simulink library "utility_lib"  (Simulink 6.3)
undefined symbols (not defined in the file): constants, MACH, quat_IC, subsref
libraries: utility_lib x28, simulink x27
settings Model: LastModifiedBy=E700252  ExtModeAutoUpdateStatusClock=off  StrictBusMsg=None

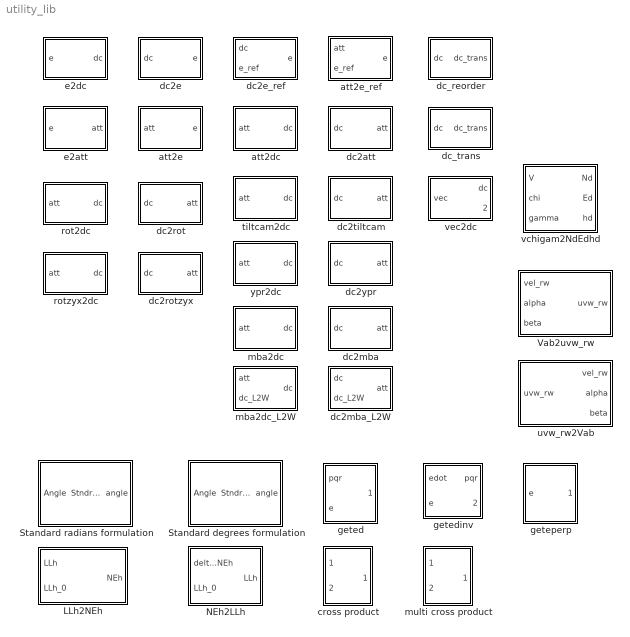
== system utility_lib ==
  LLh2NEh : Subsystem
  NEh2LLh : Subsystem
  Standard degrees formulation : Subsystem
  Standard radians formulation : Subsystem
  Vab2uvw_rw : Subsystem
  att2dc : Subsystem
  att2e : Subsystem  mask{quat_IC=quat_IC}
      mask prompts: quat_IC "quat IC"
  att2e_ref : Subsystem
  cross product : Subsystem
      mask Type: Cross Product
      mask Description: Calculates the cross product of two 3x1 vectors.
      mask Help:
      | <p>This block calculates the cross product of two 3x1 vectors, ie.</p>
      | 
      | <ul>C(1) = A(2)*B(3) - A(3)*B(2)</ul>
      | <ul>C(2) = A(3)*B(1) - A(1)*B(3)</ul>
      | <ul>C(3) = A(1)*B(2) - A(2)*B(1)</ul>
      | 
      | <p>The block inputs and output contain more than one signal as described below.</p>
      | 
      | <p><H4>Block Vector Input 1 - A</H4>
      | <ul>
      | <li>A(1)</li>
      | <li>A(2)</li>
      | <li>A(3)</li>
      | </ul>
      | </p>
      | 
      | <p><H4>Block Vector Input 2 - B</H4>
      | <ul>
      | <li>B(1)</li>
      | <li>B(2)</li>
      | <li>B(3)</li>
      | </ul>
      | </p>
      | 
      | <p><H4>Block Vector Output - Cross Product (AxB)</H4>
      | <ul>
      | <li>C(1)</li>
      | <li>C(2)</li>
      | <li>C(3)</li>
      | </ul>
      | </p>
      mask Display: disp('Cross\nProduct')
  dc2att : Subsystem
  dc2e : Subsystem  mask{quat_IC=quat_IC}
      mask prompts: quat_IC "quat IC"
  dc2e_ref : Subsystem
  dc2mba : Subsystem
  dc2mba_L2W : Subsystem
  dc2rot : Subsystem  mask{rot_order=zyx}
      mask prompts: rot_order "rot order"
      mask init:
      | try
      |     rot_def = {
      |         'zyx',[1 2 3],[1 2 3],1
      |         'yxz',[3 1 2],[2 3 1],1
      |         'xzy',[2 3 1],[3 1 2],1
      |         'xyz',[3 2 1],[3 2 1],-1
      |         'yzx',[1 3 2],[1 3 2],-1
      |         'zxy',[2 1 3],[2 1 3],-1
      |     };
      |     [tf,rot_idx] = ismember(rot_order,rot_def(:,1));
      |     rot_in_order = rot_def{rot_idx,2};
      |     rot_out_order = rot_def{rot_idx,3};
      |     rot_sign = rot_def{rot_idx,4};
      | 
      |     % set_param(gcb,'Tag',rot_order);
      | catch
      |     rethrow(lasterror)
      | end
      mask StyleString: popup(zyx|yxz|xzy|xyz|yzx|zxy)
  dc2rotzyx : Subsystem
  dc2tiltcam : Subsystem
  dc2ypr : Subsystem
  dc_reorder : Subsystem  mask{elements=[1 2 3]}
  dc_trans : Subsystem
  e2att : Subsystem
  e2dc : Subsystem
  geted : Subsystem
  getedinv : Subsystem
  geteperp : Subsystem
  mba2dc : Subsystem
  mba2dc_L2W : Subsystem
  multi cross product : Subsystem
      mask Type: Cross Product
      mask Description: Calculates the pairwise cross product of the columns of two 3xN matrices.
      mask Help:
      | <p>This block calculates the pairwise cross product of the columns of two 3xN matrices., ie.</p>
      | 
      | <ul>C(1,n) = A(2,n)*B(3,n) - A(3,n)*B(2,n)</ul>
      | <ul>C(2,n) = A(3,n)*B(1,n) - A(1,n)*B(3,n)</ul>
      | <ul>C(3,n) = A(1,n)*B(2,n) - A(2,n)*B(1,n)</ul>
      | 
      | <p>The block inputs and output contain more than one signal as described below.</p>
      | 
      | <p><H4>Block Matrix Input 1 - A(3,N)</H4></p>
      | 
      | <p><H4>Block Matrix Input 2 - B(3,N)</H4></p>
      | 
      | <p><H4>Block Matrix Output - C(3,N)</H4> </p>
      mask Display: disp('Multi\nCross\nProduct')
  rot2dc : Subsystem  mask{rot_order=zyx}
      mask prompts: rot_order "rot order"
      mask init: same as utility_lib/dc2rot
      mask StyleString: popup(zyx|yxz|xzy|xyz|yzx|zxy)
  rotzyx2dc : Subsystem
  tiltcam2dc : Subsystem
  uvw_rw2Vab : Subsystem
  vchigam2NdEdhd : Subsystem
  vec2dc : Subsystem
  ypr2dc : Subsystem

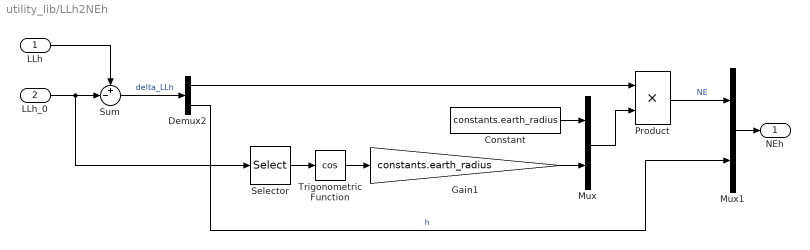
== system utility_lib/LLh2NEh ==
  LLh : Inport
  LLh_0 : Inport  Port=2
  Constant : Constant  Value=constants.earth_radius
  Demux2 : Demux  Outputs=[2 1]
  Gain1 : Gain  Gain=constants.earth_radius  SaturateOnIntegerOverflow=on
  Mux : Mux  Inputs=2
  Mux1 : Mux  Inputs=2
  Product : Product  Inputs=**  SaturateOnIntegerOverflow=on  InputSameDT=on
  Selector : Selector  InputPortWidth=3
  Sum : Sum  Inputs=+-|  SaturateOnIntegerOverflow=on  InputSameDT=on
  Trigonometric Function : Trigonometry  Operator=cos
  NEh : Outport
  wires:
  Trigonometric Function/1 -> Gain1/1
  Mux/1 -> Product/2
  LLh_0/1 -> Selector/1, Sum/2
  Demux2/2 -> Mux1/2  "h"
  Gain1/1 -> Mux/2
  Product/1 -> Mux1/1  "NE"
  Mux1/1 -> NEh/1
  Constant/1 -> Mux/1
  Selector/1 -> Trigonometric Function/1
  Sum/1 -> Demux2/1  "delta_LLh"
  Demux2/1 -> Product/1
  LLh/1 -> Sum/1

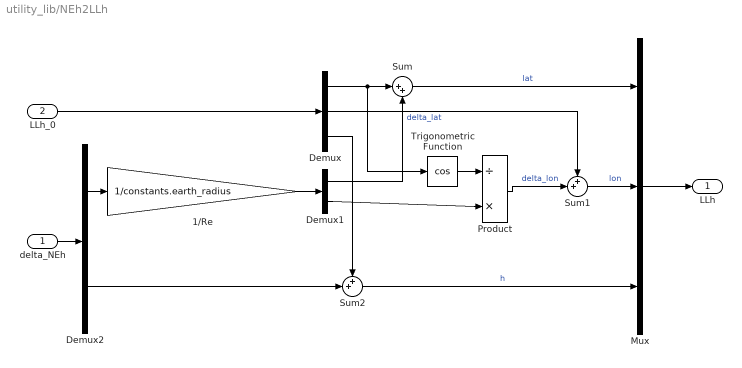
== system utility_lib/NEh2LLh ==
  delta_NEh : Inport
  LLh_0 : Inport  Port=2
  1/Re : Gain  Gain=1/constants.earth_radius  SaturateOnIntegerOverflow=on
  Demux : Demux  Outputs=3
  Demux1 : Demux  Outputs=2
  Demux2 : Demux  Outputs=[2 1]
  Mux : Mux  Inputs=3
  Product : Product  Inputs=/*  SaturateOnIntegerOverflow=on  InputSameDT=on
  Sum : Sum  Inputs=|++  SaturateOnIntegerOverflow=on  InputSameDT=on
  Sum1 : Sum  Inputs=++|  SaturateOnIntegerOverflow=on  InputSameDT=on
  Sum2 : Sum  Inputs=++|  SaturateOnIntegerOverflow=on  InputSameDT=on
  Trigonometric Function : Trigonometry  Operator=cos
  LLh : Outport
  wires:
  Mux/1 -> LLh/1
  Demux2/1 -> 1/Re/1
  Demux1/1 -> Sum/2  "delta_lat"
  Demux/1 -> Sum/1, Trigonometric Function/1
  Demux1/2 -> Product/2
  LLh_0/1 -> Demux/1
  1/Re/1 -> Demux1/1
  Sum/1 -> Mux/1  "lat"
  Trigonometric Function/1 -> Product/1
  Demux/2 -> Sum1/1
  Product/1 -> Sum1/2  "delta_lon"
  Sum1/1 -> Mux/2  "lon"
  delta_NEh/1 -> Demux2/1
  Demux2/2 -> Sum2/2
  Demux/3 -> Sum2/1
  Sum2/1 -> Mux/3  "h"

== system utility_lib/Standard degrees formulation ==
  Angle : Inport
  Constant : Constant  Value=180
  Constant1 : Constant  Value=360
  Constant2 : Constant  Value=180
  Math Function : Math  Operator=mod  SaturateOnIntegerOverflow=on
  Sum : Sum
  Sum1 : Sum  Inputs=+-
  Stndrd  angle : Outport
  wires:
  Constant2/1 -> Sum1/2
  Sum1/1 -> Stndrd  angle/1
  Math Function/1 -> Sum1/1
  Constant1/1 -> Math Function/2
  Constant/1 -> Sum/2
  Angle/1 -> Sum/1
  Sum/1 -> Math Function/1

== system utility_lib/Standard radians formulation ==
  Angle : Inport
  Constant : Constant  Value=pi
  Constant1 : Constant  Value=2*pi
  Constant2 : Constant  Value=pi
  Math Function : Math  Operator=mod  SaturateOnIntegerOverflow=on
  Sum : Sum
  Sum1 : Sum  Inputs=+-
  Stndrd  angle : Outport
  wires:
  Constant2/1 -> Sum1/2
  Sum1/1 -> Stndrd  angle/1
  Math Function/1 -> Sum1/1
  Constant1/1 -> Math Function/2
  Constant/1 -> Sum/2
  Angle/1 -> Sum/1
  Sum/1 -> Math Function/1

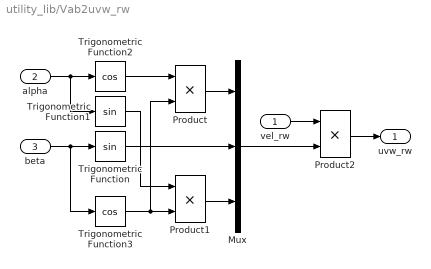
== system utility_lib/Vab2uvw_rw ==
  vel_rw : Inport
  alpha : Inport  Port=2
  beta : Inport  Port=3
  Mux : Mux  Inputs=3
  Product : Product  RndMeth=Zero
  Product1 : Product  RndMeth=Zero
  Product2 : Product  RndMeth=Zero
  Trigonometric Function : Trigonometry
  Trigonometric Function1 : Trigonometry
  Trigonometric Function2 : Trigonometry  Operator=cos
  Trigonometric Function3 : Trigonometry  Operator=cos
  uvw_rw : Outport
  wires:
  alpha/1 -> Trigonometric Function2/1, Trigonometric Function1/1
  beta/1 -> Trigonometric Function3/1, Trigonometric Function/1
  Trigonometric Function2/1 -> Product/1
  Trigonometric Function3/1 -> Product/2, Product1/2
  Trigonometric Function1/1 -> Product1/1
  Trigonometric Function/1 -> Mux/2
  Product1/1 -> Mux/3
  Product/1 -> Mux/1
  Mux/1 -> Product2/2
  vel_rw/1 -> Product2/1
  Product2/1 -> uvw_rw/1

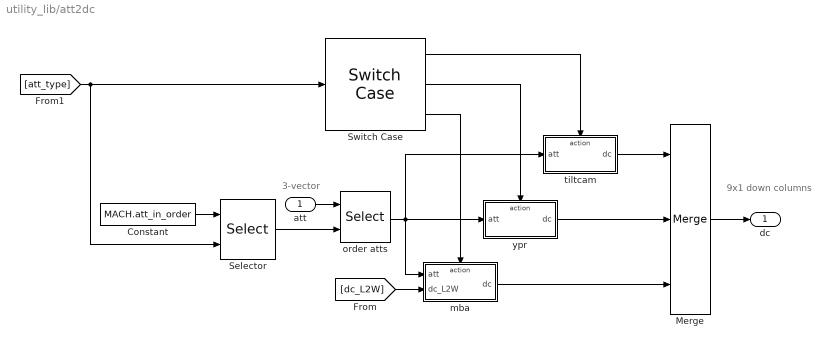
== system utility_lib/att2dc ==
  note: 3-vector
  note: 9x1
      | down columns
  att : Inport
  Constant : Constant  Value=MACH.att_in_order
  Merge : Merge  Inputs=3
  Selector : Selector  InputType=Matrix  Elements=[1 3]  RowSrc=External  Columns=-1  InputPortWidth=3
  Switch Case : SwitchCase  CaseConditions={1, [2 3], [4 5]}  CaseShowDefault=off
  mba : Subsystem  TreatAsAtomicUnit=on
  order atts : Selector  ElementSrc=External  Elements=att_order  InputPortWidth=3
  tiltcam : Subsystem  TreatAsAtomicUnit=on
  ypr : Subsystem  TreatAsAtomicUnit=on
  dc : Outport
  wires:
  order atts/1 -> ypr/1(att), tiltcam/1(att), mba/1(att)
  att/1 -> order atts/1
  Merge/1 -> dc/1
  [att_type] -> Switch Case/1, Selector/2
  tiltcam/1(dc) -> Merge/1
  ypr/1(dc) -> Merge/2
  mba/1(dc) -> Merge/3
  Switch Case/1 -> tiltcam/Action
  Switch Case/2 -> ypr/Action
  Switch Case/3 -> mba/Action
  [dc_L2W] -> mba/2(dc_L2W)
  Selector/1 -> order atts/2
  Constant/1 -> Selector/1

== system utility_lib/att2e ==
  att : Inport  PortDimensions=3
  att2dc : utility_lib/att2dc
  dc2e : utility_lib/dc2e  quat_IC=quat_IC
  e : Outport
  wires:
  att2dc/1 -> dc2e/1
  att/1 -> att2dc/1
  dc2e/1 -> e/1

== system utility_lib/att2e_ref ==
  att : Inport  PortDimensions=3
  e_ref : Inport  Port=2
  att2dc : utility_lib/att2dc
  dc2e_ref : utility_lib/dc2e_ref
  e : Outport
  wires:
  dc2e_ref/1 -> e/1
  att/1 -> att2dc/1
  att2dc/1 -> dc2e_ref/1
  e_ref/1 -> dc2e_ref/2

== system utility_lib/cross product ==
  a(1) a(2) a(3) : Inport
  b(1) b(2) b(3) : Inport  Port=2
  Product : Product  SaturateOnIntegerOverflow=on  RndMeth=Zero  InputSameDT=on
  Product1 : Product  SaturateOnIntegerOverflow=on  RndMeth=Zero  InputSameDT=on
  Selector : Selector  Elements=[2 3 1]  InputPortWidth=3
  Selector1 : Selector  Elements=[3 1 2]  InputPortWidth=3
  Selector2 : Selector  Elements=[2 3 1]  InputPortWidth=3
  Selector3 : Selector  Elements=[3 1 2]  InputPortWidth=3
  Sum : Sum  Inputs=+|-  SaturateOnIntegerOverflow=on  InputSameDT=on
  c(1) c(2) c(3) : Outport  InitialOutput=0
  wires:
  Selector3/1 -> Product1/1
  Selector2/1 -> Product1/2
  Product1/1 -> Sum/2
  Selector1/1 -> Product/2
  Product/1 -> Sum/1
  a(1) a(2) a(3)/1 -> Selector3/1, Selector/1
  Selector/1 -> Product/1
  b(1) b(2) b(3)/1 -> Selector2/1, Selector1/1
  Sum/1 -> c(1) c(2) c(3)/1

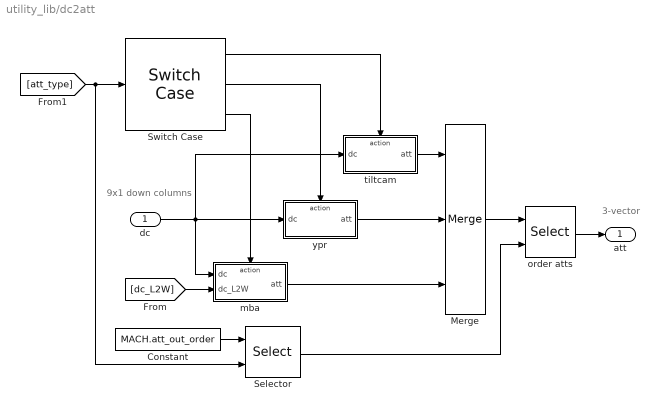
== system utility_lib/dc2att ==
  note: 9x1
      | down columns
  note: 3-vector
  dc : Inport
  Constant : Constant  Value=MACH.att_out_order
  Merge : Merge  Inputs=3
  Selector : Selector  InputType=Matrix  Elements=[1 3]  RowSrc=External  Columns=-1  InputPortWidth=3
  Switch Case : SwitchCase  CaseConditions={1, [2 3], [4 5]}  CaseShowDefault=off
  mba : Subsystem  TreatAsAtomicUnit=on
  order atts : Selector  ElementSrc=External  Elements=att_order  InputPortWidth=3
  tiltcam : Subsystem  TreatAsAtomicUnit=on
  ypr : Subsystem  TreatAsAtomicUnit=on
  att : Outport
  wires:
  [dc_L2W] -> mba/2(dc_L2W)
  Switch Case/2 -> ypr/Action
  Switch Case/1 -> tiltcam/Action
  mba/1(att) -> Merge/3
  ypr/1(att) -> Merge/2
  tiltcam/1(att) -> Merge/1
  [att_type] -> Switch Case/1, Selector/2
  Merge/1 -> order atts/1
  dc/1 -> mba/1(dc), tiltcam/1(dc), ypr/1(dc)
  order atts/1 -> att/1
  Selector/1 -> order atts/2
  Constant/1 -> Selector/1
  Switch Case/3 -> mba/Action

== system utility_lib/dc2e ==
  note: choose sign to align new
      | quaternion as closely as possible
      | in the direction of the old one.
  dc : Inport
  Unit Delay : UnitDelay  Orientation=left  X0=quat_IC  SampleTime=-1
  dc2e_ref : utility_lib/dc2e_ref
  e : Outport
  wires:
  dc/1 -> dc2e_ref/1
  dc2e_ref/1 -> e/1, Unit Delay/1
  Unit Delay/1 -> dc2e_ref/2

== system utility_lib/dc2e_ref ==
  note: choose sign to align new
      | quaternion as closely as possible
      | in the direction of the reference input
  dc : Inport
  e_ref : Inport  Port=2
  Compute quat : Subsystem
  Dot Product : simulink/Math Operations/Dot Product  InputSameDT=on  OutDataType=sfix(16)  OutScaling=2^-10  DoSatur=off
  Gain : Gain  Gain=-1  SaturateOnIntegerOverflow=on
  Switch : Switch  SaturateOnIntegerOverflow=on
  e : Outport
  wires:
  e_ref/1 -> Dot Product/2
  Gain/1 -> Switch/3
  Dot Product/1 -> Switch/2
  Compute quat/1(e) -> Gain/1, Switch/1, Dot Product/1
  Switch/1 -> e/1
  dc/1 -> Compute quat/1(dc)

== system utility_lib/dc2mba ==
  dc : Inport
  Gain1 : Gain  Gain=[1 1 -1]
  Math Function : Math  Operator=transpose  SaturateOnIntegerOverflow=on
  Product : Product  Multiplication=Matrix(*)  RndMeth=Zero
  Reshape1 : simulink/Math Operations/Reshape  OutputDimensionality=1-D array  OutputDimensions=[3 3]
  Reshape2 : simulink/Math Operations/Reshape  OutputDimensionality=Customize  OutputDimensions=[3 3]
  Reshape3 : simulink/Math Operations/Reshape  OutputDimensionality=Customize  OutputDimensions=[3 3]
  dc2rot : utility_lib/dc2rot  rot_order=xzy
  att : Outport
  wires:
  Reshape1/1 -> dc2rot/1
  Math Function/1 -> Product/2
  Reshape2/1 -> Math Function/1
  Reshape3/1 -> Product/1
  dc/1 -> Reshape3/1
  Product/1 -> Reshape1/1
  [dc_L2W] -> Reshape2/1
  Gain1/1 -> att/1
  dc2rot/1 -> Gain1/1

== system utility_lib/dc2mba_L2W ==
  dc : Inport
  dc_L2W : Inport  Port=2
  Gain1 : Gain  Gain=[1 1 -1]
  Math Function : Math  Operator=transpose  SaturateOnIntegerOverflow=on
  Product : Product  Multiplication=Matrix(*)  RndMeth=Zero
  Reshape1 : simulink/Math Operations/Reshape  OutputDimensionality=1-D array  OutputDimensions=[3 3]
  Reshape2 : simulink/Math Operations/Reshape  OutputDimensionality=Customize  OutputDimensions=[3 3]
  Reshape3 : simulink/Math Operations/Reshape  OutputDimensionality=Customize  OutputDimensions=[3 3]
  dc2rot : utility_lib/dc2rot  rot_order=xzy
  att : Outport
  wires:
  dc2rot/1 -> Gain1/1
  Gain1/1 -> att/1
  dc_L2W/1 -> Reshape2/1
  Product/1 -> Reshape1/1
  dc/1 -> Reshape3/1
  Reshape3/1 -> Product/1
  Reshape2/1 -> Math Function/1
  Math Function/1 -> Product/2
  Reshape1/1 -> dc2rot/1

== system utility_lib/dc2rot ==
  note: 3-vector OUT
  note: 9x1
      | down columns
  dc : Inport
  Gain : Gain  Gain=rot_sign
  Selector1 : Selector  Elements=rot_out_order  InputPortWidth=3
  dc2rotzyx : utility_lib/dc2rotzyx
  dc_reorder : utility_lib/dc_reorder  elements=rot_in_order
  att : Outport
  wires:
  Selector1/1 -> Gain/1
  dc2rotzyx/1 -> Selector1/1
  dc_reorder/1 -> dc2rotzyx/1
  dc/1 -> dc_reorder/1
  Gain/1 -> att/1

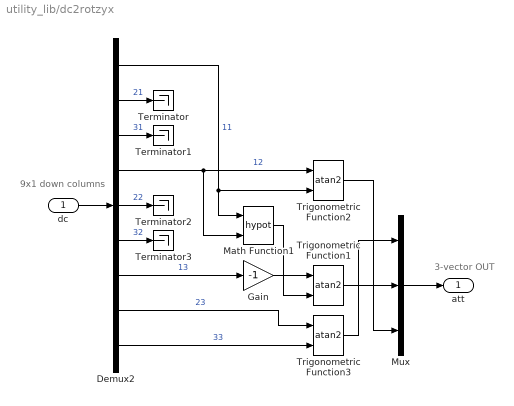
== system utility_lib/dc2rotzyx ==
  note: 3-vector OUT
  note: 9x1
      | down columns
  dc : Inport
  Demux2 : Demux  Outputs=9
  Gain : Gain  Gain=-1  SaturateOnIntegerOverflow=on
  Math Function1 : Math  Operator=hypot  SaturateOnIntegerOverflow=on
  Mux : Mux  Inputs=3
  Terminator{,1..3} (4 alike) : Terminator
  Trigonometric Function1 : Trigonometry  Operator=atan2
  Trigonometric Function2 : Trigonometry  Operator=atan2
  Trigonometric Function3 : Trigonometry  Operator=atan2
  att : Outport
  wires:
  Demux2/9 -> Trigonometric Function3/2  "33"
  Demux2/8 -> Trigonometric Function3/1  "23"
  Demux2/6 -> Terminator3/1  "32"
  Demux2/5 -> Terminator2/1  "22"
  Demux2/4 -> Trigonometric Function2/1, Math Function1/2  "12"
  Demux2/3 -> Terminator1/1  "31"
  Demux2/2 -> Terminator/1  "21"
  Demux2/1 -> Trigonometric Function2/2, Math Function1/1  "11"
  dc/1 -> Demux2/1
  Trigonometric Function3/1 -> Mux/1
  Trigonometric Function2/1 -> Mux/3
  Trigonometric Function1/1 -> Mux/2
  Mux/1 -> att/1
  Demux2/7 -> Gain/1  "13"
  Gain/1 -> Trigonometric Function1/1
  Math Function1/1 -> Trigonometric Function1/2

== system utility_lib/dc2tiltcam ==
  note: 9x1
      | down columns
  dc : Inport
  Gain : Gain  Gain=MACH.body2vert  Multiplication=Matrix(K*u)
  Reshape : simulink/Math Operations/Reshape  OutputDimensionality=Customize  OutputDimensions=[3 3]
  Reshape1 : simulink/Math Operations/Reshape  OutputDimensionality=1-D array  OutputDimensions=[3 3]
  dc2rot : utility_lib/dc2rot  rot_order=xyz
  att : Outport
  wires:
  dc/1 -> Reshape/1
  dc2rot/1 -> att/1
  Gain/1 -> Reshape1/1
  Reshape/1 -> Gain/1
  Reshape1/1 -> dc2rot/1

== system utility_lib/dc2ypr ==
  note: 9x1
      | down columns
  dc : Inport
  Gain : Gain  Gain=MACH.body2horz  Multiplication=Matrix(K*u)
  Reshape : simulink/Math Operations/Reshape  OutputDimensionality=Customize  OutputDimensions=[3 3]
  Reshape1 : simulink/Math Operations/Reshape  OutputDimensionality=1-D array  OutputDimensions=[3 3]
  dc2rot : utility_lib/dc2rot  rot_order=zyx
  att : Outport
  wires:
  Reshape1/1 -> dc2rot/1
  Reshape/1 -> Gain/1
  Gain/1 -> Reshape1/1
  dc2rot/1 -> att/1
  dc/1 -> Reshape/1

== system utility_lib/dc_reorder ==
  dc : Inport
  Selector : Selector  Elements=reshape(subsref(reshape(1:9,3,3),struct('type','()','subs',{{elements,elements}})),1,9)  InputPortWidth=9
  dc_trans : Outport
  wires:
  Selector/1 -> dc_trans/1
  dc/1 -> Selector/1

== system utility_lib/dc_trans ==
  dc : Inport
  Selector : Selector  Elements=reshape(reshape(1:9,3,3)',1,9)  InputPortWidth=9
  dc_trans : Outport
  wires:
  dc/1 -> Selector/1
  Selector/1 -> dc_trans/1

== system utility_lib/e2att ==
  e : Inport
  dc2att : utility_lib/dc2att
  e2dc : utility_lib/e2dc
  att : Outport
  wires:
  dc2att/1 -> att/1
  e2dc/1 -> dc2att/1
  e/1 -> e2dc/1

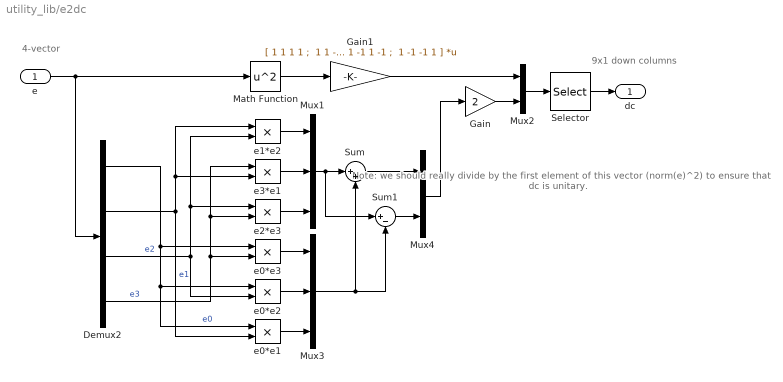
== system utility_lib/e2dc ==
  note: 4-vector
  note: 9x1
      | down columns
  note: Note: we should really divide by
      | the first element of this vector
      | (norm(e)^2) to ensure that dc
      | is unitary.
  e : Inport
  Demux2 : Demux
  Gain : Gain  Gain=2
  Gain1 : Gain  Gain="[ 1 1 1 1 ;  1 1 -1 -1 ;  1 -1 1 -1 ;  1 -1 -1 1 ]"  Multiplication=Matrix(K*u)
  Math Function : Math  Operator=square  SaturateOnIntegerOverflow=on
  Mux1 : Mux  Inputs=3
  Mux2 : Mux  Inputs=2
  Mux3 : Mux  Inputs=3
  Mux4 : Mux  Inputs=2
  Selector : Selector  Elements=[2 8 6 5 3 10 9 7 4]  InputPortWidth=10
  Sum : Sum  Inputs=|++
  Sum1 : Sum  Inputs=|+-
  e0*e1 : Product  SaturateOnIntegerOverflow=on  InputSameDT=on
  e0*e2 : Product  SaturateOnIntegerOverflow=on  InputSameDT=on
  e0*e3 : Product  SaturateOnIntegerOverflow=on  InputSameDT=on
  e1*e2 : Product  SaturateOnIntegerOverflow=on  InputSameDT=on
  e2*e3 : Product  SaturateOnIntegerOverflow=on  InputSameDT=on
  e3*e1 : Product  SaturateOnIntegerOverflow=on  InputSameDT=on
  dc : Outport
  wires:
  e/1 -> Demux2/1, Math Function/1
  Gain1/1 -> Mux2/1
  Mux4/1 -> Gain/1
  Demux2/1 -> e0*e3/1, e0*e2/1, e0*e1/1  "e0"
  Demux2/2 -> e0*e1/2, e1*e2/1, e3*e1/2  "e1"
  Demux2/3 -> e2*e3/1, e1*e2/2, e0*e2/2  "e2"
  Demux2/4 -> e0*e3/2, e3*e1/1, e2*e3/2  "e3"
  Math Function/1 -> Gain1/1
  e1*e2/1 -> Mux1/1
  e3*e1/1 -> Mux1/2
  e2*e3/1 -> Mux1/3
  e0*e3/1 -> Mux3/1
  e0*e2/1 -> Mux3/2
  e0*e1/1 -> Mux3/3
  Mux2/1 -> Selector/1
  Selector/1 -> dc/1
  Gain/1 -> Mux2/2
  Mux1/1 -> Sum/1, Sum1/1
  Mux3/1 -> Sum/2, Sum1/2
  Sum/1 -> Mux4/1
  Sum1/1 -> Mux4/2

== system utility_lib/geted ==
  pqr : Inport
  e : Inport  Port=2
  Gain4 : Gain  Gain=0.5  SaturateOnIntegerOverflow=on
  Product : Product  Inputs=**  Multiplication=Matrix(*)  SaturateOnIntegerOverflow=on  InputSameDT=on
  geteperp : utility_lib/geteperp
  e_dot : Outport
  wires:
  geteperp/1 -> Product/1
  e/1 -> geteperp/1
  pqr/1 -> Product/2
  Product/1 -> Gain4/1
  Gain4/1 -> e_dot/1

== system utility_lib/getedinv ==
  note: get p, q, r from e0d, e1d, e2d, e3d, e0, e1, e2, e3
      |
      | this is a dynamic inverse routine it does not solve the equations exactly
      |  unless ed satisfies the quaternion constraint
  edot : Inport
  e : Inport  Port=2
  Gain : Gain  Gain=2
  Math Function : Math  Operator=transpose  SaturateOnIntegerOverflow=on
  Product : Product  Multiplication=Matrix(*)  RndMeth=Zero
  geteperp : utility_lib/geteperp
  pqr : Outport
  e_perp : Outport  Port=2
  wires:
  edot/1 -> Product/2
  geteperp/1 -> Math Function/1, e_perp/1
  Gain/1 -> Product/1
  Product/1 -> pqr/1
  Math Function/1 -> Gain/1
  e/1 -> geteperp/1

== system utility_lib/geteperp ==
  e : Inport
  Gain1 : Gain  Gain=[-1 1 1 -1]  SaturateOnIntegerOverflow=on
  Gain2 : Gain  Gain=[-1 -1 1 1]  SaturateOnIntegerOverflow=on
  Gain3 : Gain  Gain=[-1 1 -1 1]  SaturateOnIntegerOverflow=on
  Matrix Concatenation : simulink/Math Operations/Matrix Concatenation  numInports=3  catMethod=Horizontal
  Reshape : simulink/Math Operations/Reshape  OutputDimensionality=Column vector  OutputDimensions=[1,1]
  Reshape1 : simulink/Math Operations/Reshape  OutputDimensionality=Column vector  OutputDimensions=[1,1]
  Reshape2 : simulink/Math Operations/Reshape  OutputDimensionality=Column vector  OutputDimensions=[1,1]
  Selector : Selector  Elements=[2 1 4 3]  InputPortWidth=4
  Selector1 : Selector  Elements=[3 4 1 2]  InputPortWidth=4
  Selector2 : Selector  Elements=[4 3 2 1]  InputPortWidth=4
  e_perp : Outport
  wires:
  Selector2/1 -> Gain3/1
  Selector1/1 -> Gain2/1
  Selector/1 -> Gain1/1
  Gain1/1 -> Reshape/1
  Gain3/1 -> Reshape2/1
  Gain2/1 -> Reshape1/1
  Matrix Concatenation/1 -> e_perp/1
  e/1 -> Selector2/1, Selector1/1, Selector/1
  Reshape/1 -> Matrix Concatenation/1
  Reshape1/1 -> Matrix Concatenation/2
  Reshape2/1 -> Matrix Concatenation/3

== system utility_lib/mba2dc ==
  att : Inport
  Gain1 : Gain  Gain=[1 1 -1]
  Product : Product  Multiplication=Matrix(*)  RndMeth=Zero
  Reshape1 : simulink/Math Operations/Reshape  OutputDimensionality=Customize  OutputDimensions=[3 3]
  Reshape2 : simulink/Math Operations/Reshape  OutputDimensionality=Customize  OutputDimensions=[3 3]
  Reshape3 : simulink/Math Operations/Reshape  OutputDimensionality=1-D array  OutputDimensions=[3 3]
  rot2dc : utility_lib/rot2dc  rot_order=xzy
  dc : Outport
  wires:
  att/1 -> Gain1/1
  Gain1/1 -> rot2dc/1
  rot2dc/1 -> Reshape1/1
  [dc_L2W] -> Reshape2/1
  Product/1 -> Reshape3/1
  Reshape1/1 -> Product/1
  Reshape2/1 -> Product/2
  Reshape3/1 -> dc/1

== system utility_lib/mba2dc_L2W ==
  att : Inport
  dc_L2W : Inport  Port=2
  Gain1 : Gain  Gain=[1 1 -1]
  Product : Product  Multiplication=Matrix(*)  RndMeth=Zero
  Reshape1 : simulink/Math Operations/Reshape  OutputDimensionality=Customize  OutputDimensions=[3 3]
  Reshape2 : simulink/Math Operations/Reshape  OutputDimensionality=Customize  OutputDimensions=[3 3]
  Reshape3 : simulink/Math Operations/Reshape  OutputDimensionality=1-D array  OutputDimensions=[3 3]
  rot2dc : utility_lib/rot2dc  rot_order=xzy
  dc : Outport
  wires:
  Reshape3/1 -> dc/1
  Reshape2/1 -> Product/2
  Reshape1/1 -> Product/1
  Product/1 -> Reshape3/1
  dc_L2W/1 -> Reshape2/1
  rot2dc/1 -> Reshape1/1
  Gain1/1 -> rot2dc/1
  att/1 -> Gain1/1

== system utility_lib/multi cross product ==
  a(1) a(2) a(3) : Inport
  b(1) b(2) b(3) : Inport  Port=2
  Product : Product  SaturateOnIntegerOverflow=on  RndMeth=Zero  InputSameDT=on
  Product1 : Product  SaturateOnIntegerOverflow=on  RndMeth=Zero  InputSameDT=on
  Selector4 : Selector  InputType=Matrix  Elements=[1 3]  Rows=[2 3 1]  Columns=-1  InputPortWidth=3
  Selector5 : Selector  InputType=Matrix  Elements=[1 3]  Rows=[2 3 1]  Columns=-1  InputPortWidth=3
  Selector6 : Selector  InputType=Matrix  Elements=[1 3]  Rows=[3 1 2]  Columns=-1  InputPortWidth=3
  Selector7 : Selector  InputType=Matrix  Elements=[1 3]  Rows=[3 1 2]  Columns=-1  InputPortWidth=3
  Sum : Sum  Inputs=+|-  SaturateOnIntegerOverflow=on  InputSameDT=on
  c(1) c(2) c(3) : Outport  InitialOutput=0
  wires:
  Sum/1 -> c(1) c(2) c(3)/1
  b(1) b(2) b(3)/1 -> Selector7/1, Selector5/1
  Selector4/1 -> Product/1
  a(1) a(2) a(3)/1 -> Selector4/1, Selector6/1
  Product/1 -> Sum/1
  Selector7/1 -> Product/2
  Product1/1 -> Sum/2
  Selector6/1 -> Product1/1
  Selector5/1 -> Product1/2

== system utility_lib/rot2dc ==
  note: 9x1
      | down columns
  note: 3-vector
  att : Inport
  Gain : Gain  Gain=rot_sign
  Selector1 : Selector  Elements=rot_in_order  InputPortWidth=3
  dc_reorder : utility_lib/dc_reorder  elements=rot_out_order
  rotzyx2dc : utility_lib/rotzyx2dc
  dc : Outport
  wires:
  Selector1/1 -> rotzyx2dc/1
  rotzyx2dc/1 -> dc_reorder/1
  Gain/1 -> Selector1/1
  dc_reorder/1 -> dc/1
  att/1 -> Gain/1

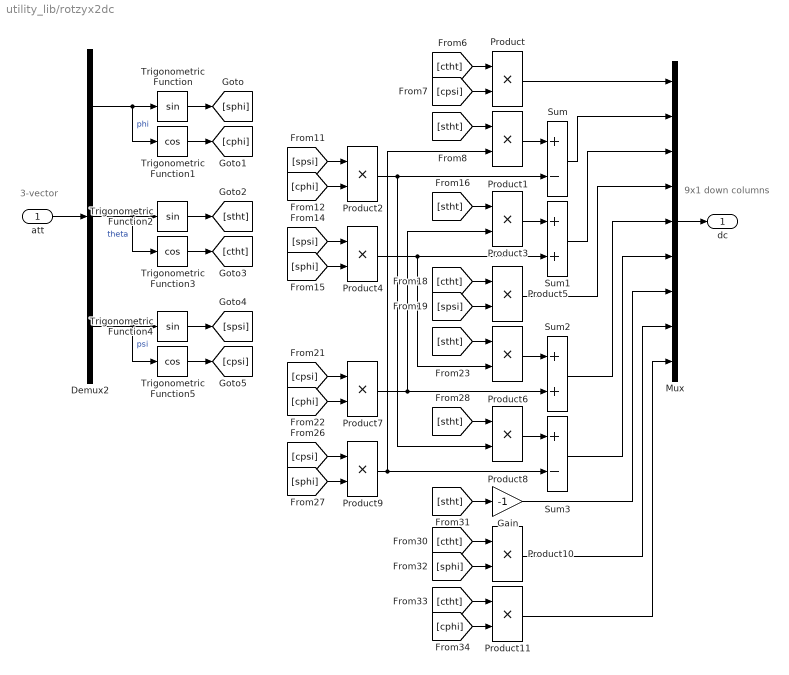
== system utility_lib/rotzyx2dc ==
  note: 9x1
      | down columns
  note: 3-vector
  att : Inport
  Demux2 : Demux  Outputs=3
  Gain : Gain  Gain=-1  SaturateOnIntegerOverflow=on
  Mux : Mux  Inputs=9
  Product{,1..11} (12 alike) : Product  SaturateOnIntegerOverflow=on  InputSameDT=on
  Sum : Sum  Inputs=+-  SaturateOnIntegerOverflow=on  InputSameDT=on
  Sum1 : Sum  SaturateOnIntegerOverflow=on  InputSameDT=on
  Sum2 : Sum  SaturateOnIntegerOverflow=on  InputSameDT=on
  Sum3 : Sum  Inputs=+-  SaturateOnIntegerOverflow=on  InputSameDT=on
  Trigonometric Function : Trigonometry
  Trigonometric Function1 : Trigonometry  Operator=cos
  Trigonometric Function2 : Trigonometry
  Trigonometric Function3 : Trigonometry  Operator=cos
  Trigonometric Function4 : Trigonometry
  Trigonometric Function5 : Trigonometry  Operator=cos
  dc : Outport
  wires:
  Mux/1 -> dc/1
  att/1 -> Demux2/1
  Demux2/1 -> Trigonometric Function/1, Trigonometric Function1/1  "phi"
  Demux2/2 -> Trigonometric Function2/1, Trigonometric Function3/1  "theta"
  Demux2/3 -> Trigonometric Function4/1, Trigonometric Function5/1  "psi"
  Product1/1 -> Sum/1
  Product2/1 -> Sum/2, Product8/2
  Trigonometric Function/1 -> [sphi]
  Trigonometric Function1/1 -> [cphi]
  Trigonometric Function2/1 -> [stht]
  Trigonometric Function3/1 -> [ctht]
  Trigonometric Function4/1 -> [spsi]
  Trigonometric Function5/1 -> [cpsi]
  [ctht] -> Product/1
  [cpsi] -> Product/2
  [stht] -> Product1/1
  [spsi] -> Product2/1
  Product3/1 -> Sum1/1
  Product4/1 -> Sum1/2, Product6/2
  [stht] -> Product3/1
  [spsi] -> Product4/1
  [sphi] -> Product4/2
  [ctht] -> Product5/1
  [spsi] -> Product5/2
  Product6/1 -> Sum2/1
  Product7/1 -> Sum2/2, Product3/2
  [stht] -> Product6/1
  [cpsi] -> Product7/1
  [cphi] -> Product7/2
  Product8/1 -> Sum3/1
  Product9/1 -> Sum3/2, Product1/2
  [stht] -> Product8/1
  [cpsi] -> Product9/1
  [stht] -> Gain/1
  [ctht] -> Product11/1
  Product/1 -> Mux/1
  Sum/1 -> Mux/2
  Sum1/1 -> Mux/3
  Product5/1 -> Mux/4
  Sum2/1 -> Mux/5
  Sum3/1 -> Mux/6
  Gain/1 -> Mux/7
  Product10/1 -> Mux/8
  Product11/1 -> Mux/9
  [cphi] -> Product2/2
  [sphi] -> Product9/2
  [cphi] -> Product11/2
  [ctht] -> Product10/1
  [sphi] -> Product10/2

== system utility_lib/tiltcam2dc ==
  note: 3-vector
  note: 9x1
      | down columns
  att : Inport
  Gain : Gain  Gain=MACH.vert2body  Multiplication=Matrix(K*u)
  Reshape : simulink/Math Operations/Reshape  OutputDimensionality=Customize  OutputDimensions=[3 3]
  Reshape1 : simulink/Math Operations/Reshape  OutputDimensionality=1-D array  OutputDimensions=[3 3]
  rot2dc : utility_lib/rot2dc  rot_order=xyz
  dc : Outport
  wires:
  att/1 -> rot2dc/1
  Gain/1 -> Reshape1/1
  rot2dc/1 -> Reshape/1
  Reshape/1 -> Gain/1
  Reshape1/1 -> dc/1

== system utility_lib/uvw_rw2Vab ==
  uvw_rw : Inport
  Demux : Demux  Outputs=3
  Math Function : Math  Operator=hypot  SaturateOnIntegerOverflow=on
  Math Function1 : Math  Operator=hypot  SaturateOnIntegerOverflow=on
  Trigonometric Function1 : Trigonometry  Operator=atan2
  Trigonometric Function2 : Trigonometry  Operator=atan2
  vel_rw : Outport
  alpha : Outport  Port=2
  beta : Outport  Port=3
  wires:
  Demux/3 -> Math Function/2, Trigonometric Function2/1
  Demux/1 -> Math Function/1, Trigonometric Function2/2
  Demux/2 -> Trigonometric Function1/1, Math Function1/2
  Math Function/1 -> Trigonometric Function1/2, Math Function1/1
  uvw_rw/1 -> Demux/1  "uvw_rw"
  Math Function1/1 -> vel_rw/1
  Trigonometric Function2/1 -> alpha/1
  Trigonometric Function1/1 -> beta/1

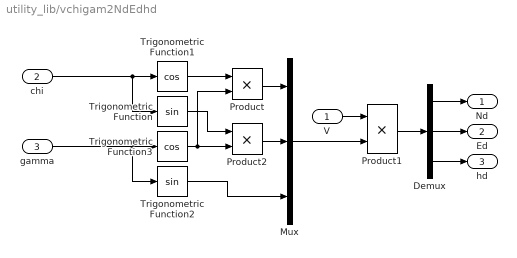
== system utility_lib/vchigam2NdEdhd ==
  V : Inport
  chi : Inport  Port=2
  gamma : Inport  Port=3
  Demux : Demux  Outputs=3
  Mux : Mux  Inputs=3
  Product : Product  RndMeth=Zero
  Product1 : Product  RndMeth=Zero
  Product2 : Product  RndMeth=Zero
  Trigonometric Function : Trigonometry
  Trigonometric Function1 : Trigonometry  Operator=cos
  Trigonometric Function2 : Trigonometry
  Trigonometric Function3 : Trigonometry  Operator=cos
  Nd : Outport
  Ed : Outport  Port=2
  hd : Outport  Port=3
  wires:
  chi/1 -> Trigonometric Function/1, Trigonometric Function1/1
  gamma/1 -> Trigonometric Function2/1, Trigonometric Function3/1
  Trigonometric Function1/1 -> Product/1
  Trigonometric Function2/1 -> Mux/3
  Trigonometric Function3/1 -> Product/2, Product2/2
  Trigonometric Function/1 -> Product2/1
  Product/1 -> Mux/1
  Product2/1 -> Mux/2
  Mux/1 -> Product1/2
  V/1 -> Product1/1
  Product1/1 -> Demux/1
  Demux/1 -> Nd/1
  Demux/2 -> Ed/1
  Demux/3 -> hd/1

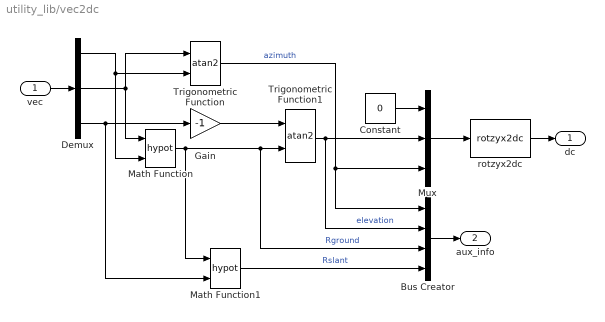
== system utility_lib/vec2dc ==
  vec : Inport
  Bus Creator : BusCreator
  Constant : Constant  Value=0
  Demux : Demux  Outputs=3
  Gain : Gain  Gain=-1
  Math Function : Math  Operator=hypot  SaturateOnIntegerOverflow=on
  Math Function1 : Math  Operator=hypot  SaturateOnIntegerOverflow=on
  Mux : Mux  Inputs=3
  Trigonometric Function : Trigonometry  Operator=atan2
  Trigonometric Function1 : Trigonometry  Operator=atan2
  rotzyx2dc : utility_lib/rotzyx2dc
  dc : Outport
  aux_info : Outport  Port=2
  wires:
  rotzyx2dc/1 -> dc/1
  vec/1 -> Demux/1
  Demux/1 -> Trigonometric Function/2, Math Function/2
  Demux/2 -> Trigonometric Function/1, Math Function/1
  Demux/3 -> Gain/1, Math Function1/2
  Gain/1 -> Trigonometric Function1/1
  Math Function/1 -> Trigonometric Function1/2, Bus Creator/3, Math Function1/1  "Rground"
  Constant/1 -> Mux/1
  Trigonometric Function1/1 -> Mux/2, Bus Creator/2  "elevation"
  Trigonometric Function/1 -> Mux/3, Bus Creator/1  "azimuth"
  Mux/1 -> rotzyx2dc/1
  Bus Creator/1 -> aux_info/1
  Math Function1/1 -> Bus Creator/4  "Rslant"

== system utility_lib/ypr2dc ==
  note: 9x1
      | down columns
  note: 3-vector
  att : Inport
  Gain : Gain  Gain=MACH.horz2body  Multiplication=Matrix(K*u)
  Reshape : simulink/Math Operations/Reshape  OutputDimensionality=Customize  OutputDimensions=[3 3]
  Reshape1 : simulink/Math Operations/Reshape  OutputDimensionality=1-D array  OutputDimensions=[3 3]
  rot2dc : utility_lib/rot2dc  rot_order=zyx
  dc : Outport
  wires:
  Reshape1/1 -> dc/1
  Reshape/1 -> Gain/1
  rot2dc/1 -> Reshape/1
  Gain/1 -> Reshape1/1
  att/1 -> rot2dc/1

== system utility_lib/att2dc/mba ==
  att : Inport
  dc_L2W : Inport  Port=2
  Action Port : ActionPort  ActionType=case
  mba2dc_L2W : utility_lib/mba2dc_L2W
  dc : Outport
  wires:
  att/1 -> mba2dc_L2W/1
  mba2dc_L2W/1 -> dc/1
  dc_L2W/1 -> mba2dc_L2W/2

== system utility_lib/att2dc/tiltcam ==
  att : Inport
  Action Port : ActionPort  ActionType=case
  tiltcam2dc : utility_lib/tiltcam2dc
  dc : Outport
  wires:
  att/1 -> tiltcam2dc/1
  tiltcam2dc/1 -> dc/1

== system utility_lib/att2dc/ypr ==
  att : Inport
  Action Port : ActionPort  ActionType=case
  ypr2dc : utility_lib/ypr2dc
  dc : Outport
  wires:
  att/1 -> ypr2dc/1
  ypr2dc/1 -> dc/1

== system utility_lib/dc2att/mba ==
  dc : Inport
  dc_L2W : Inport  Port=2
  Action Port : ActionPort  ActionType=case
  dc2mba_L2W : utility_lib/dc2mba_L2W
  att : Outport
  wires:
  dc_L2W/1 -> dc2mba_L2W/2
  dc2mba_L2W/1 -> att/1
  dc/1 -> dc2mba_L2W/1

== system utility_lib/dc2att/tiltcam ==
  dc : Inport
  Action Port : ActionPort  ActionType=case
  dc2tiltcam : utility_lib/dc2tiltcam
  att : Outport
  wires:
  dc2tiltcam/1 -> att/1
  dc/1 -> dc2tiltcam/1

== system utility_lib/dc2att/ypr ==
  dc : Inport
  Action Port : ActionPort  ActionType=case
  dc2ypr : utility_lib/dc2ypr
  att : Outport
  wires:
  dc2ypr/1 -> att/1
  dc/1 -> dc2ypr/1

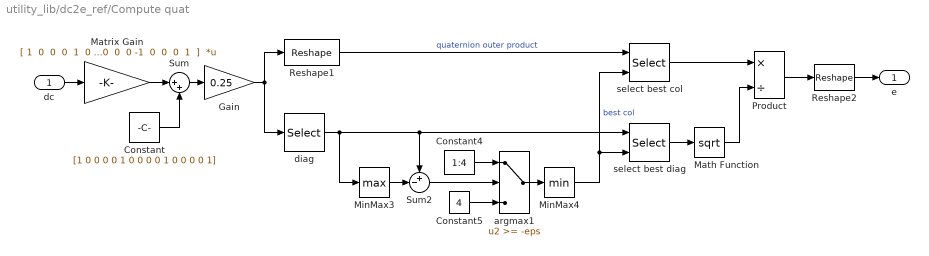
== system utility_lib/dc2e_ref/Compute quat ==
  dc : Inport
  Constant : Constant  Value=[1 0 0 0 0 1 0 0 0 0 1 0 0 0 0 1]
  Constant4 : Constant  Value=1:4
  Constant5 : Constant  Value=4
  Gain : Gain  Gain=0.25  SaturateOnIntegerOverflow=on
  Math Function : Math  Operator=sqrt  SaturateOnIntegerOverflow=on
  Matrix Gain : Gain  Gain="[ 1  0  0  0  1  0  0  0  1 ; 0  0  0  0  0 -1  0  1  0 ; 0  0  1  0  0  0 -1  0  0 ; 0 -1  0  1  0  0  0  0  0 ; 0  0  0  0  0 -1  0  1  0 ; 1  0  0  0 -1  0  0  0 -1 ; 0  1  0  1  0  0  0  0  0 ; 0  0  1  0  0  0  1  0  0 ; 0  0  1  0  0  0 -1  0  0 ; 0  1  0  1  0  0  0  0  0 ; -1  0  0  0  1  0  0  0 -1 ; 0  0  0  0  0  1  0  1  0 ; 0 -1  0  1  0  0  0  0  0 ; 0  0  1  0  0  0  1  0  0 ; 0  0  0  0  0  1  0  1  0 ; -1  0  0  0 -1  0  0  0  1  ]"  Multiplication=Matrix(K*u)  SaturateOnIntegerOverflow=on
  MinMax3 : MinMax  Function=max  SaturateOnIntegerOverflow=on  InputSameDT=on
  MinMax4 : MinMax  SaturateOnIntegerOverflow=on  InputSameDT=on
  Product : Product  Inputs=*/  SaturateOnIntegerOverflow=on
  Reshape1 : simulink/Math Operations/Reshape  OutputDimensionality=Customize  OutputDimensions=[4,4]
  Reshape2 : simulink/Math Operations/Reshape  OutputDimensionality=1-D array  OutputDimensions=[4,4]
  Sum : Sum  Inputs=|++  SaturateOnIntegerOverflow=on
  Sum2 : Sum  Inputs=+-|  SaturateOnIntegerOverflow=on
  argmax1 : Switch  Threshold=-eps  SaturateOnIntegerOverflow=on
  diag : Selector  Elements=[1 6 11 16]  InputPortWidth=16
  select best col : Selector  InputType=Matrix  ElementSrc=External  Elements=-1  Rows=-1  ColumnSrc=External  InputPortWidth=3
  select best diag : Selector  ElementSrc=External  Elements=-1  Rows=-1  ColumnSrc=External  InputPortWidth=4
  e : Outport
  wires:
  dc/1 -> Matrix Gain/1
  Matrix Gain/1 -> Sum/1
  Constant/1 -> Sum/2
  Sum/1 -> Gain/1
  Gain/1 -> diag/1, Reshape1/1
  diag/1 -> MinMax3/1, select best diag/1, Sum2/1
  Reshape1/1 -> select best col/1  "quaternion outer product"
  Reshape2/1 -> e/1
  Sum2/1 -> argmax1/2
  Constant4/1 -> argmax1/1
  Constant5/1 -> argmax1/3
  argmax1/1 -> MinMax4/1
  MinMax4/1 -> select best col/2, select best diag/2  "best col"
  select best diag/1 -> Math Function/1
  select best col/1 -> Product/1
  Math Function/1 -> Product/2
  Product/1 -> Reshape2/1
  MinMax3/1 -> Sum2/2
